simulink model "TCS"  (R2023a)
settings: Solver=VariableStepAuto  StartTime=0.0  StopTime=50  RelTol=1e-3
libraries: slpidlib x1
settings Model: Creator=ibaad  LastModifiedBy=ibaad
settings DebuggingCC: AlgebraicLoopMsg=none

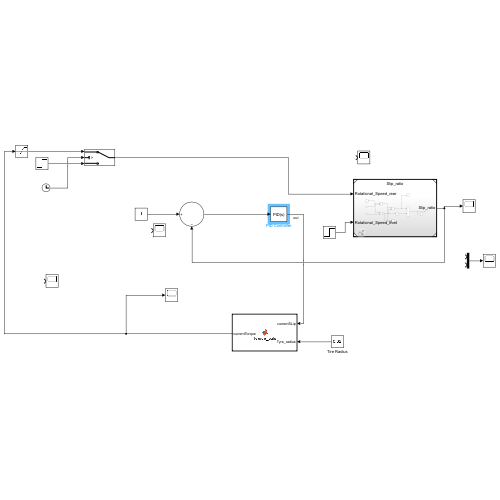
[thumbnail: Simulink's stored preview of the top-level diagram]
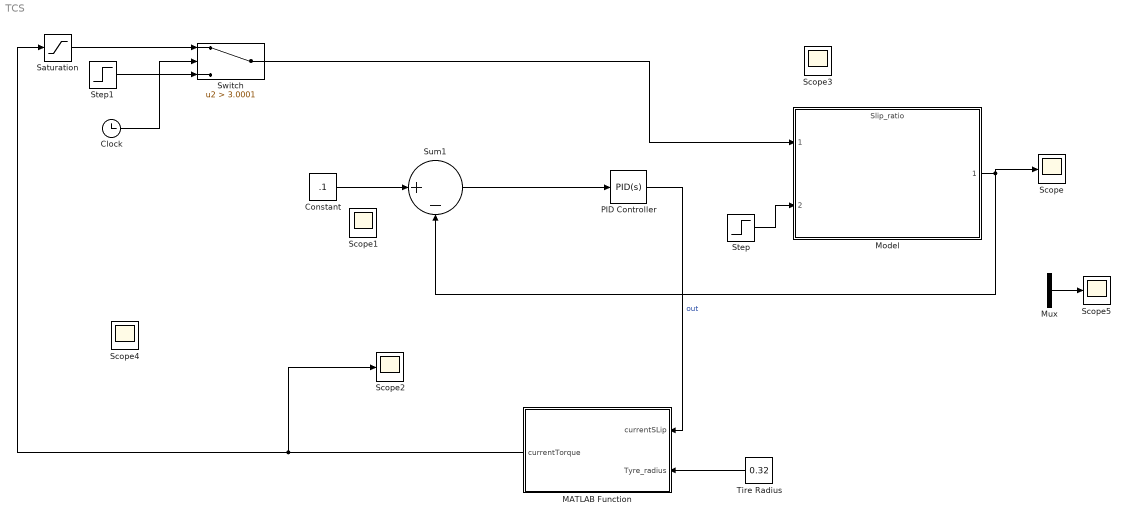
== system TCS ==
  Clock : Clock
  Constant : Constant  Value=.1
  MATLAB Function : MATLAB Function  TreatAsAtomicUnit=on
  Model : ModelReference  ModelNameDialog=Slip_ratio.slx  SimulationMode=Normal  ModelReferenceVersion=1.5
  Mux : Mux  Inputs=2
  PID Controller : slpidlib/PID Controller  Controller=PID  Form=Parallel  TimeDomain=Continuous-time  UseExternalTs=off  SampleTime=-1  IntegratorMethod=Forward Euler  FilterMethod=Forward Euler  ControllerParametersSource=internal  P=1000  I=150  UseKiTs=off  D=0.0025  N=100  UseFilter=on  TunerSelectOption=Transfer Function Based (PID Tuner App)  InitialConditionSource=internal  InitialConditionForIntegrator=0  InitialConditionForFilter=0  DifferentiatorICPrevScaledInput=0  ExternalReset=none  TrackingMode=off  Kt=1  LimitOutput=off  SatLimitsSource=internal  UpperSaturationLimit=inf  LowerSaturationLimit=-inf  LinearizeAsGain=on  AntiWindupMode=none  Kb=1  LimitIntegrator=off  UpperIntegratorSaturationLimit=inf  LowerIntegratorSaturationLimit=-inf  POutMin=[]  POutMax=[]  IOutMin=[]  IOutMax=[]  DOutMin=[]  DOutMax=[]  NOutMin=[]  NOutMax=[]  SumOutMin=[]  SumOutMax=[]  SaturationOutMin=[]  SaturationOutMax=[]  PParamMin=[]  PParamMax=[]  IParamMin=[]  IParamMax=[]  DParamMin=[]  DParamMax=[]  NParamMin=[]  NParamMax=[]  KbParamMin=[]  KbParamMax=[]  KtParamMin=[]  KtParamMax=[]  KbOutMin=[]  KbOutMax=[]  KtOutMin=[]  KtOutMax=[]  IntegratorOutMin=[]  IntegratorOutMax=[]  FilterOutMin=[]  FilterOutMax=[]  SumI1OutMin=[]  SumI1OutMax=[]  SumI2OutMin=[]  SumI2OutMax=[]  SumI3OutMin=[]  SumI3OutMax=[]  SumI4OutMin=[]  SumI4OutMax=[]  SumDOutMin=[]  SumDOutMax=[]  DifferentiatorOutMin=[]  DifferentiatorOutMax=[]  FilterDiffOutCoefMin=[]  FilterDiffOutCoefMax=[]  ReciprocalOutMin=[]  ReciprocalOutMax=[]  SumDenOutMin=[]  SumDenOutMax=[]  SumNumOutMin=[]  SumNumOutMax=[]  DivideOutMin=[]  DivideOutMax=[]  UdiffTsProdOutMin=[]  UdiffTsProdOutMax=[]  NTsProdOutMin=[]  NTsProdOutMax=[]  UintegralTsProdOutMin=[]  UintegralTsProdOutMax=[]  UngainTsProdOutMin=[]  UngainTsProdOutMax=[]  ClampingZeroOutDataTypeStr=Inherit: Inherit via back propagation  ClampingZeroOutMin=[]  ClampingZeroOutMax=[]  FilterDenConstantOutDataTypeStr=Inherit: Inherit via back propagation  FilterDenConstantOutMin=[]  FilterDenConstantOutMax=[]  PCopyOutDataTypeStr=Inherit: Inherit via back propagation  PCopyOutMin=[]  PCopyOutMax=[]  NCopyOutDataTypeStr=Inherit: Inherit via back propagation  NCopyOutMin=[]  NCopyOutMax=[]  IntegratorContinuousStateAttributes=''  IntegratorStateMustResolveToSignalObject=off  IntegratorRTWStateStorageClass=Auto  FilterContinuousStateAttributes=''  FilterStateMustResolveToSignalObject=off  FilterRTWStateStorageClass=Auto  ParallelPVariant=InternalParameters  IdealPVariant=Disabled  IVariant=InternalParameters  DVariant=InternalParameters  IntegratorVariant=Continuous  SatVariant=Disabled  AWVariant=Passthrough  PCopyVariant=Disabled  TRVariant=Disabled  FdbkBlocksVariant=Forward  IdealPFdbkVariant=Disabled  SatFdbkVariant=Disabled  DerivativeFilterVariant=ContFilter  NVariant=InternalParameters  NCopyVariant=Disabled  FilterICVariant=InternalICsFilter  IntegratorICVariant=InternalICs  ExternalResetVariant=Disabled  TRSumVariant=Passthrough  SumFdbkVariant=Disabled  SumVariant=Sum_PID  TsampFilterVariant=InternalTs  TsampNgainVariant=Passthrough  TsampIntegralVariant=Disabled_SignalSpec  ExternalSaturationOutDataTypeStr=Inherit: Same as second input
  Saturation : Saturate  UpperLimit=320  LowerLimit=1
  Scope{,1..5} (6 alike) : Scope
  Step : Step  Time=3  After=175  SampleTime=0
  Step1 : Step  Time=3  After=200  SampleTime=0
  Sum1 : Sum  Inputs=|+-
  Switch : Switch  Criteria=u2 > Threshold  Threshold=3.0001  SaturateOnIntegerOverflow=off  InputSameDT=off
  Tire Radius : Constant  Value=0.32
  wires:
  Saturation/1 -> Switch/1
  Sum1/1 -> PID Controller/1
  Tire Radius/1 -> MATLAB Function/2(Tyre_radius)
  MATLAB Function/1(currentTorque) -> Scope2/1, Saturation/1
  Step/1 -> Model/2
  Mux/1 -> Scope5/1
  Constant/1 -> Sum1/1
  Step1/1 -> Switch/3
  Switch/1 -> Model/1
  Model/1 -> Scope/1, Sum1/2
  PID Controller/1 -> MATLAB Function/1(currentSLip)  "out"
  Clock/1 -> Switch/2

== matlab function TCS/MATLAB Function ==
  data: currentTorque output; currentSLip input; Tyre_radius input
function currentTorque = Torque_calc(currentSLip, Tyre_radius)
    % TCS_ACTIVE Summary of this function goes here

    e = exp(1); % Mathematical constant e
    % Friction curve as a function of slip ratio
    c1 = 1.2801; % Coef for dry asphalt
    c2 = 23.99; % Coef for dry asphalt
    c3 = 0.52; % Coef for dry asphalt
    Fn = 1350; % Normal force on one tire
    

 %   plot(slip_ratios, fricCoef); % Plot the entire array
 %   xlabel("Slip Ratio");
 %   ylabel("Longitudinal Friction Coefficient");
 %   title("Friction Coefficient vs. Slip Ratio Curve");
 %   grid on;% Optionally, turn the grid on for better readability


    fricCoef = c1 * (1 - exp(-c2 * currentSLip)) - c3 * currentSLip;
    currentTorque = ((fricCoef * Fn) * Tyre_radius);
end
